simulink model "Stage1"  (R2016a)
settings: Solver=VariableStepAuto  SolverMode=SingleTasking  StartTime=0.0  StopTime=10.0  RelTol=1e-3
PreLoadFcn:
  | System.m
model workspace: external: MATLAB File C:\Users\darre\Desktop\Measurements\Project simulation Matlab\System.m (data not in the file)
values from neighbouring files (symbols this model uses):
  den1s = [1 (1/(R2*C1)+1/(R1*C1)) 1/(R1*C1*R2*C2)]    [System.m]
  den2s = [1 (1/(R2*C1)+1/(R1*C1)) 1/(R1*C1*R2*C2)]    [System.m]
  den3s = [1 (1/(R2*C1)+1/(R1*C1)) 1/(R1*C1*R2*C2)]    [System.m]
  den4s = [1 (1/(R2*C1)+1/(R1*C1)) 1/(R1*C1*R2*C2)]    [System.m]
  num1s = [1/(R1*C1*R2*C2)]    [System.m]
  num2s = [1/(R1*C1*R2*C2)]    [System.m]
  num3s = [1/(R1*C1*R2*C2)]    [System.m]
  num4s = [1/(R1*C1*R2*C2)]    [System.m]
libraries: simulink x1
settings Model: Creator=darre  LastModifiedBy=darre
settings DataIOCC: LimitDataPoints=on  SaveOutput=off  SaveTime=off
settings OptimizationCC: BlockReduction=off  BooleanDataType=off
settings DebuggingCC: SaveWithParameterizedLinksMsg=none  UnderspecifiedInitializationDetection=Classic  MergeDetectMultiDrivingBlocksExec=none  SignalResolutionControl=TryResolveAllWithWarning  AllowSymbolicDim=off
settings HardwareCC: TargetUnknown=on

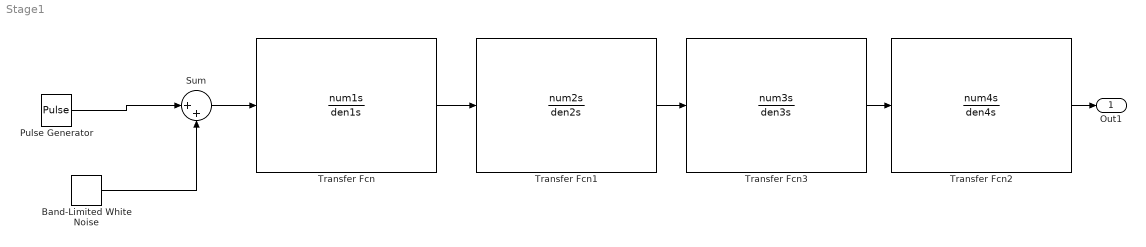
== system Stage1 ==
  Band-Limited White Noise : simulink/Sources/Band-Limited White Noise  Cov=[0.000000001]  Ts=0.00001  seed=[230341]
  Pulse Generator : DiscretePulseGenerator  PulseType=Time based  Amplitude=3.3  Period=0.01  PulseWidth=50
  Sum : Sum  Inputs=|++
  Transfer Fcn : TransferFcn  Numerator=num1s  Denominator=den1s
  Transfer Fcn1 : TransferFcn  Numerator=num2s  Denominator=den2s
  Transfer Fcn2 : TransferFcn  Numerator=num4s  Denominator=den4s
  Transfer Fcn3 : TransferFcn  Numerator=num3s  Denominator=den3s
  Out1 : Outport
  wires:
  Transfer Fcn/1 -> Transfer Fcn1/1
  Sum/1 -> Transfer Fcn/1
  Transfer Fcn1/1 -> Transfer Fcn3/1
  Transfer Fcn3/1 -> Transfer Fcn2/1
  Transfer Fcn2/1 -> Out1/1
  Pulse Generator/1 -> Sum/1
  Band-Limited White Noise/1 -> Sum/2
